simulink model "circuito"  (Simulink 7.7)
settings: Solver=ode3  StartTime=0.0  StopTime=1  FixedStep=2e-5  RelTol=1e-3
undefined symbols (not defined in the file): get
libraries: commchan3 x1, commsink2 x1, commrandsrc2 x1
settings Model: Creator=ctu  LastModifiedBy=ctu

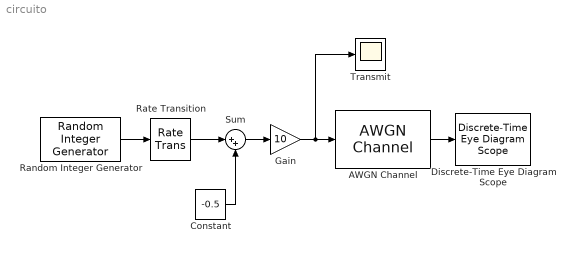
== system circuito ==
  AWGN Channel : commchan3/AWGN Channel  SystemSampleTime=-1  InputProcessing=Inherited (this choice will be removed - see release notes)  seed=randseed  noiseMode=Variance from mask  EbNodB=10  EsNodB=10  SNRdB=10  bitsPerSym=1  Ps=1  Tsym=1  variance=6
  Constant : Constant  Value=-0.5
  Discrete-Time Eye Diagram Scope : commsink2/Discrete-Time Eye Diagram Scope  Tag=EyeDiagram  SystemSampleTime=-1  sampPerSymb=50  offsetEye=0  symbPerTrace=2  numTraces=50  numNewFrames=50  LineMarkers=none  LineStyles=-  LineColors=b  dupPoints=on  fading=on  render=on  AxisGrid=on  yMin=-8  yMax=7  inphaseLabel=In-phase Amplitude  quadratureLabel=Quadrature Amplitude  openScopeAtSimStart=on  dispDiagram=In-phase and Quadrature  FrameNumber=off  FigPos=get(0,'defaultfigureposition');  figTitle=Eye Diagram  block_type_=eye  numLinesMax=8
  Gain : Gain  Gain=10
  Random Integer Generator : commrandsrc2/Random Integer Generator  SystemSampleTime=-1  mul=2  seed=randseed  Ts=1e-3  frameBased=off  sampPerFrame=1  orient=on  outDataType=double
  Rate Transition : RateTransition  OutPortSampleTime=2e-5
  Sum : Sum  Inputs=|++
  Transmit : Scope
  wires:
  Constant/1 -> Sum/2
  Rate Transition/1 -> Sum/1
  Random Integer Generator/1 -> Rate Transition/1
  Sum/1 -> Gain/1
  AWGN Channel/1 -> Discrete-Time Eye Diagram Scope/1
  Gain/1 -> AWGN Channel/1, Transmit/1
